simulink model "platform_model"  (R2024b)
settings: Solver=VariableStepAuto  StartTime=0.0  StopTime=60  RelTol=1e-3
values from neighbouring files (symbols this model uses):
  A_s = [1 0 0 ... (first row only)    [main.m]
  E_b_0 = [0; 0; 0]    [main.m]
  I_ws = blkdiag(I_ws, I_wi)    [main.m]
  J = I_b + A_s*Inrt_s*A_s' + A_t*Inrt_t*A_t' + A_g*Inrt_g*A_g'    [main.m]
  k_d = (J.*2*zeta*w_n)    [main.m]
  k_p = (2*J.*w_n^2)    [main.m]
  T = [0;0;0]    [main.m]
  w_b_0 = [0; 0; 0]    [main.m]
settings Model: Creator=Jacob  LastModifiedBy=Jacob

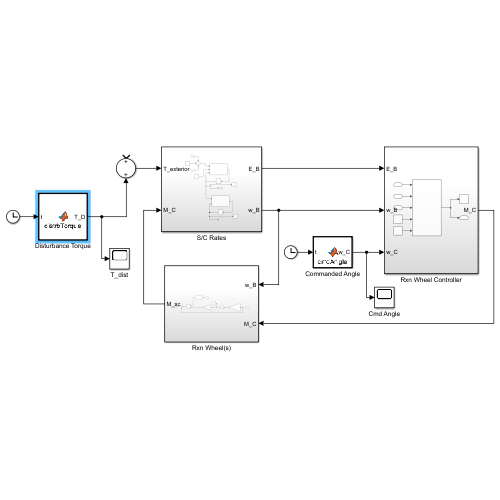
[thumbnail: Simulink's stored preview of the top-level diagram]
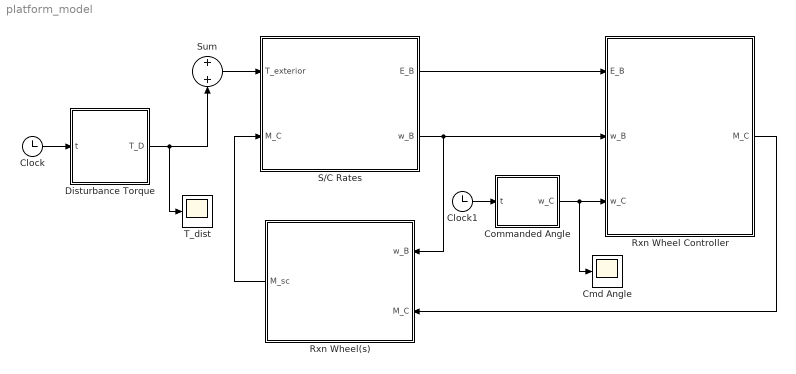
== system platform_model ==
  Clock : Clock
  Clock1 : Clock
  Cmd Angle : Scope
  Commanded Angle : MATLAB Function  TreatAsAtomicUnit=on
  Disturbance Torque : MATLAB Function  TreatAsAtomicUnit=on
  Rxn Wheel Controller : Subsystem
  Rxn Wheel(s) : Subsystem
  S/C Rates : Subsystem
  Sum : Sum  Inputs=+|+  InputSameDT=on
  T_dist : Scope
  wires:
  S/C Rates/2(w_B) -> Rxn Wheel(s)/1(w_B), Rxn Wheel Controller/2(w_B)
  Rxn Wheel Controller/1(M_C) -> Rxn Wheel(s)/2(M_C)
  Rxn Wheel(s)/1(M_sc) -> S/C Rates/2(M_C)
  Clock1/1 -> Commanded Angle/1(t)
  Commanded Angle/1(w_C) -> Cmd Angle/1, Rxn Wheel Controller/3(w_C)
  Clock/1 -> Disturbance Torque/1(t)
  S/C Rates/1(E_B) -> Rxn Wheel Controller/1(E_B)
  Sum/1 -> S/C Rates/1(T_exterior)
  Disturbance Torque/1(T_D) -> T_dist/1, Sum/2

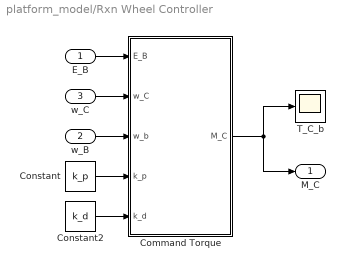
== system platform_model/Rxn Wheel Controller ==
  E_B : Inport
  w_B : Inport  Port=2
  w_C : Inport  Port=3
  Command Torque : MATLAB Function  TreatAsAtomicUnit=on
  Constant : Constant  Value=k_p
  Constant2 : Constant  Value=k_d
  T_C_b : Scope
  M_C : Outport
  wires:
  w_B/1 -> Command Torque/3(w_b)
  Constant/1 -> Command Torque/4(k_p)
  Constant2/1 -> Command Torque/5(k_d)
  Command Torque/1(M_C) -> T_C_b/1, M_C/1
  w_C/1 -> Command Torque/2(w_C)
  E_B/1 -> Command Torque/1(E_B)

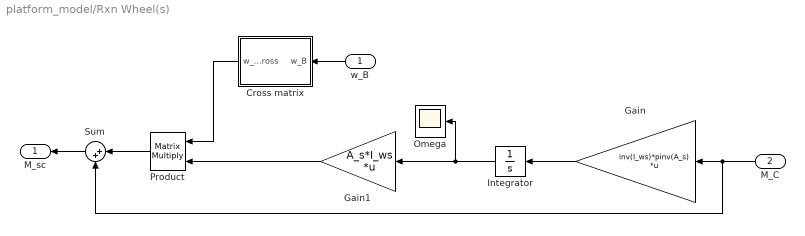
== system platform_model/Rxn Wheel(s) ==
  w_B : Inport
  M_C : Inport  Port=2
  Cross matrix : MATLAB Function  TreatAsAtomicUnit=on
  Gain : Gain  Gain=inv(I_ws)*pinv(A_s)  Multiplication=Matrix(K*u)
  Gain1 : Gain  Gain=A_s*I_ws  Multiplication=Matrix(K*u) (u vector)
  Integrator : Integrator
  Omega : Scope
  Product : Product  Multiplication=Matrix(*)
  Sum : Sum  Inputs=|++
  M_sc : Outport
  wires:
  M_C/1 -> Sum/2, Gain/1
  Gain1/1 -> Product/2
  Integrator/1 -> Omega/1, Gain1/1
  Product/1 -> Sum/1
  Sum/1 -> M_sc/1
  Gain/1 -> Integrator/1
  w_B/1 -> Cross matrix/1(w_B)
  Cross matrix/1(w_B_cross) -> Product/1

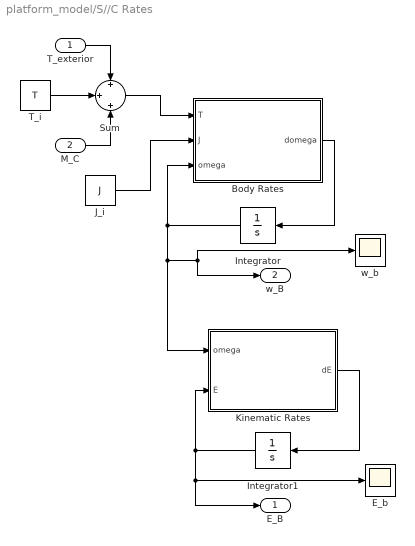
== system platform_model/S//C Rates ==
  T_exterior : Inport
  M_C : Inport  Port=2
  Body Rates : MATLAB Function  TreatAsAtomicUnit=on
  E_b : Scope
  Integrator : Integrator  InitialCondition=w_b_0
  Integrator1 : Integrator  InitialCondition=E_b_0
  J_i : Constant  Value=J
  Kinematic Rates : MATLAB Function  TreatAsAtomicUnit=on
  Sum : Sum  Inputs=+|+|+  InputSameDT=on
  T_i : Constant  Value=T
  w_b : Scope
  E_B : Outport
  w_B : Outport  Port=2
  wires:
  J_i/1 -> Body Rates/2(J)
  Body Rates/1(domega) -> Integrator/1
  Sum/1 -> Body Rates/1(T)
  Kinematic Rates/1(dE) -> Integrator1/1
  T_exterior/1 -> Sum/1
  T_i/1 -> Sum/2
  M_C/1 -> Sum/3
  Integrator/1 -> Body Rates/3(omega), w_b/1, w_B/1, Kinematic Rates/1(omega)
  Integrator1/1 -> E_B/1, E_b/1, Kinematic Rates/2(E)

== matlab function platform_model/Rxn Wheel Controller/Command Torque ==
  data: E_B input; w_C input; M_C output; w_b input; k_p input; k_d input
function M_C  = cmdTorque(E_B, w_C, w_b, k_p, k_d)
% Function computes command torque
%#codegen

% Command torque calc
M_C = -k_p*E_B - k_d*(w_b - w_C); % N-m

== matlab function platform_model/S//C Rates/Body Rates ==
  data: T input; J input; omega input; domega output
function domega = dynamics(T, J, omega)
% Function computes the derivative of the angular velocity
%#codegen

domega = J \ (T - cross(omega, (J*omega)));

== matlab function platform_model/S//C Rates/Kinematic Rates ==
  data: omega input; E input; dE output
function dE  = kinematics(omega, E)
% Function computes the Euler and Quaternion derivatives
%#codegen

% Calculating the derivative of the Euler Angle components
            
% Euler rates
phi   = E(1);
theta = E(2);

LBI = 1/cos(theta)*[cos(theta) sin(phi)*sin(theta)  cos(phi)*sin(theta);
                     0         cos(phi)*cos(theta) -sin(phi)*cos(theta);
                     0         sin(phi)            cos(phi)];
    
dE = LBI*omega;

== matlab function platform_model/Disturbance Torque ==
  data: t input; T_D output
function T_D = distrbTorque(t)
% Function computes the simulated disturbance torque
%#codegen

if t >= 10 && t < 15
    T_D = [-4; 0; 0]*10e-3;
elseif t >= 15 && t < 25
    T_D = [-4; -4; 0]*10e-3;
elseif t >= 25 && t < 30
    T_D = [0; -4; 0]*10e-3;
else
    T_D = [0; 0; 0];
end

== matlab function platform_model/Rxn Wheel(s)/Cross matrix ==
  data: w_B input; w_B_cross output
function w_B_cross = vectCross(w_B)

w_B_cross = vectCross(w_B);

== matlab function platform_model/Commanded Angle ==
  data: t input; w_C output
function w_C = cmdAngle(t)
% Function applies a command angle at different times
%#codegen

if t >= 10 && t < 15
    w_C = [15*(pi/180); 0;0];
elseif t >= 15 && t < 25
    w_C = [15*(pi/180); 15*(pi/180); -15*(pi/180)];
elseif t >= 25 && t < 30
    w_C = [0; 15*(pi/180);0];
else
    w_C = [0; 0; 0];
end
